simulink model "Vis_CSGO_T_L_NM"  (R2017a)
settings: Solver=FixedStepDiscrete  StartTime=0.0  StopTime=inf  FixedStep=1/250  RelTol=1e-3  EnableMultiTasking=on
StopFcn:
  | AutoStartBatchData=load('session1.mat');AutoStartBatchData=AutoStartBatchData.y;run('AEP_P300_Evaluation')
model workspace (MAT data in the model file):
  cfg_native : struct (value not decoded)
  en_add_channels = 127
  host_ip = 2130706433
  host_port = 50223
  local_ip = 2130706433
  local_port = 50224
  num_en_channels = 32
  num_samples = 4
  sample_rate = 250
  serial_number = 'NR-2018.09.02'
undefined symbols (not defined in the file): groupMap, NR
libraries: gtecHighspeedLib x9, simulink x3, gNautilusLib x1
settings Model: Creator=Holzner  LastModifiedBy=user
settings DataIOCC: LimitDataPoints=on  SaveFormat=Array
settings OptimizationCC: LifeSpan=inf
settings DebuggingCC: UnderspecifiedInitializationDetection=Classic  MergeDetectMultiDrivingBlocksExec=none  SolverPrmCheckMsg=warning  FrameProcessingCompatibilityMsg=none  StateNameClashWarn=warning  SFUnexpectedBacktrackingDiag=warning  SFNoUnconditionalDefaultTransitionDiag=warning  SFExecutionAtInitializationDiag=none
settings HardwareCC: ProdBitPerPointer=32  ProdBitPerSizeT=32  ProdBitPerPtrDiffT=32  ProdLargestAtomicFloat=None  ProdIntDivRoundTo=Undefined  ProdEndianess=Unspecified  ProdWordSize=32  ProdHWDeviceType=32-bit Generic
settings ModelReferenceCC: PropagateSignalLabelsOutOfModel=off
settings GRTTargetCC: TargetLangStandard=C89/C90 (ANSI)  GeneratePreprocessorConditionals=Disable all
settings ConfigComp: CovMetricSettings=dw  CovHtmlReporting=on  CovSaveCumulativeToWorkspaceVar=on  CovSaveSingleToWorkspaceVar=on  CovExternalEMLEnable=off  CovSFcnEnable=off

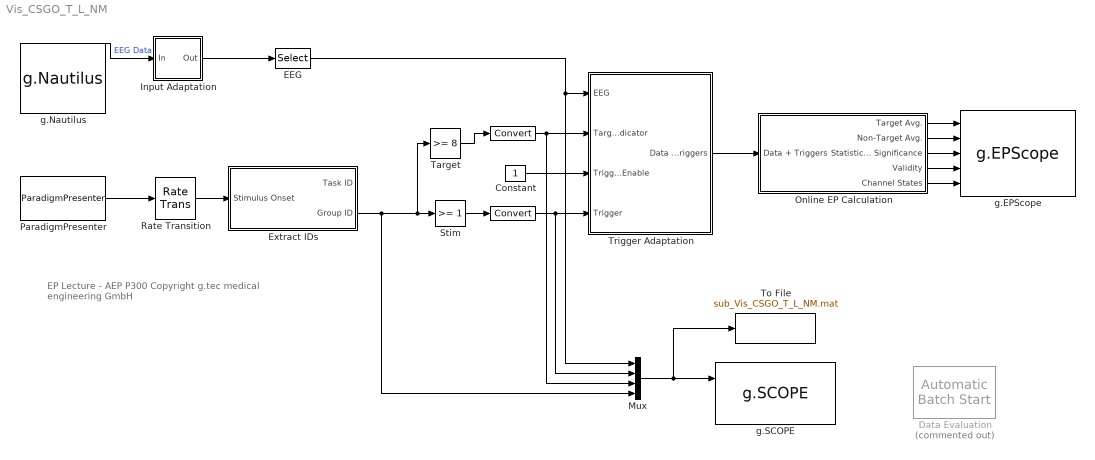
== system Vis_CSGO_T_L_NM ==
  note: EP Lecture - AEP P300
      | Copyright g.tec medical engineering GmbH
  " " : DataTypeConversion
  "  " : DataTypeConversion
  Constant : Constant  SampleTime=-1
  Data Evaluation : gtecHighspeedLib/Automatic  Batch Start  Commented=on  batch2start='AEP_P300_Evaluation'  nameToFileBlock=empty
      settings: SourceProductName=g.tec Highspeed Library
  EEG : Selector  InputPortWidth=32  IndexOptions=Index vector (dialog)  Indices=[1:32]  OutputSizes=1
  Extract IDs : Subsystem
  Input Adaptation : Subsystem
  Mux : Mux
  Online EP Calculation : Subsystem  mask(Online EP Calculation){data_ch_count=32}
      mask prompts: data_ch_count "Number of data channels:"
      mask help:
      | Calculates the target and non-target average of the incoming data and performs statistical significance analysis of target and non-target frames.
      | The data coming in must contain 'Number of data channel' data channels, trigger IDs and target triggers.
  ParadigmPresenter : gtecHighspeedLib/ParadigmPresenter  Priority=2  bufferSize=000001  sampleRateOrig=000250  stimQuantizationUs=002000  paradigmRootFolder=C:\Users\user.T440_IT\Documents\gtec\gtecHS\Examples_can_be_changed\ParadigmPresenter\Sk_CSGO_exp_xml  logLevel=1  paradigmFiles=\Demo\ParadigmPresenterDemo.xml
      settings: SourceProductName=g.tec Highspeed Library
  Rate Transition : RateTransition
  Stim : simulink/Logic and Bit Operations/Compare To Constant  relop=>=  const=1  OutDataTypeStr=boolean
  Target : simulink/Logic and Bit Operations/Compare To Constant  relop=>=  const=8  OutDataTypeStr=boolean
  To File : ToFile  Filename=sub_Vis_CSGO_T_L_NM.mat  MatrixName=y
  Trigger Adaptation : Subsystem
  g.EPScope : gtecHighspeedLib/g.EPScope
      settings: SourceProductName=g.tec Highspeed Library
  g.Nautilus : gNautilusLib/g.Nautilus  Tag=g.Nautilus  Description=Operates a g.Nautilus device and provides acquired data on its outputs.  sample_rate=250  local_ip=2130706433  local_port=50224  host_ip=2130706433  host_port=50223  serial_number=NR-2018.09.02  num_samples=4  num_en_channels=32  add_channels=127
      settings: SourceProductName=g.Nautilus
  g.SCOPE : gtecHighspeedLib/g.SCOPE
      settings: SourceProductName=g.tec Highspeed Library
  wires:
  EEG/1 -> Mux/1, Trigger Adaptation/1(EEG)
  Input Adaptation/1(Out) -> EEG/1
  g.Nautilus/1 -> Input Adaptation/1(In)  "EEG Data"
  Mux/1 -> To File/1, g.SCOPE/1
  Online EP Calculation/1(Target Avg.) -> g.EPScope/1
  Online EP Calculation/2(Non-Target Avg.) -> g.EPScope/2
  Online EP Calculation/3(Statistical Significance) -> g.EPScope/3
  Online EP Calculation/4(Validity) -> g.EPScope/4
  Online EP Calculation/5(Channel States) -> g.EPScope/5
  Trigger Adaptation/1(Data + Triggers) -> Online EP Calculation/1(Data + Triggers)
  ParadigmPresenter/1 -> Rate Transition/1
  Rate Transition/1 -> Extract IDs/1(Stimulus Onset)
  Extract IDs/2(Group ID) -> Target/1, Stim/1, Mux/4
  Target/1 -> " "/1
  Constant/1 -> Trigger Adaptation/3(Trigger Enable)
  "  "/1 -> Mux/2, Trigger Adaptation/4(Trigger)
  Stim/1 -> "  "/1
  " "/1 -> Trigger Adaptation/2(Target Indicator), Mux/3

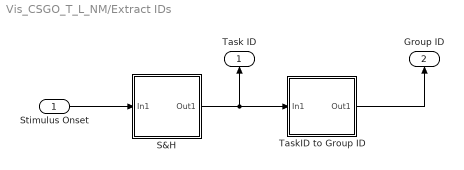
== system Vis_CSGO_T_L_NM/Extract IDs ==
  Stimulus Onset : Inport
  S&H : Subsystem
  TaskID to Group ID : Subsystem  InitFcn=|
      | try
      |   taskInfo = evalin('base','taskInfo');
      |   groupMap = taskInfo.Group;
      | catch ME
      |   clear ME;
      |   error('No paradigm loaded!');
      | end
  Task ID : Outport
  Group ID : Outport  Port=2
  wires:
  TaskID to Group ID/1(Out1) -> Group ID/1
  S&H/1(Out1) -> TaskID to Group ID/1(In1), Task ID/1
  Stimulus Onset/1 -> S&H/1(In1)

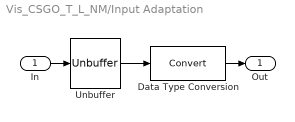
== system Vis_CSGO_T_L_NM/Input Adaptation ==
  In : Inport
  Data Type Conversion : DataTypeConversion
  Unbuffer : Unbuffer
  Out : Outport
  wires:
  In/1 -> Unbuffer/1
  Unbuffer/1 -> Data Type Conversion/1
  Data Type Conversion/1 -> Out/1

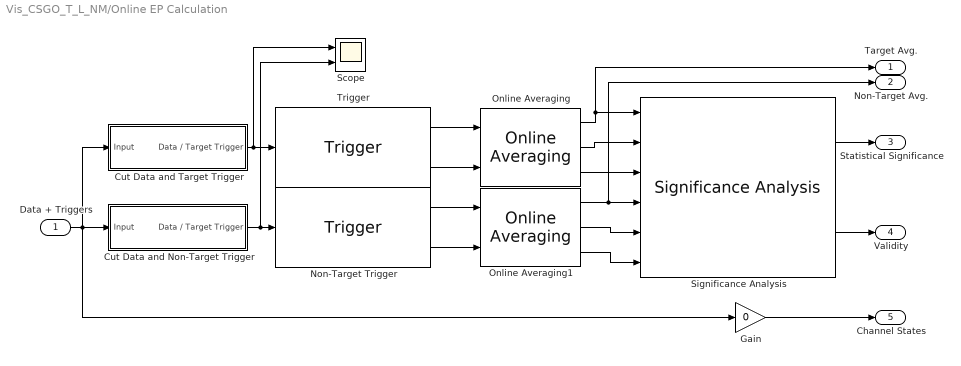
== system Vis_CSGO_T_L_NM/Online EP Calculation ==
  Data + Triggers : Inport
  Cut Data and Non-Target Trigger : Subsystem
  Cut Data and Target Trigger : Subsystem
  Gain : Gain  Gain=0
  Non-Target Trigger : gtecHighspeedLib/Trigger  trigchan=9  edge_select=RISING  edge=0  treshold=1  ext_treshold=off  windowsize=0.7  pretrigger=-0.1  sampletime=1/250  validity_select=STANDARD (global validity flag for all channels)  validity=0
      settings: SourceProductName=g.tec Highspeed Library
  Online Averaging : gtecHighspeedLib/Online Averaging  mode_select=1 - average all data  mode=0  window=10  add_std=on  do_baseline_correction=off  baseline_interval=[0 0]  sampletime=1/250
      settings: SourceProductName=g.tec Highspeed Library
  Online Averaging1 : gtecHighspeedLib/Online Averaging  mode_select=1 - average all data  mode=0  window=10  add_std=on  do_baseline_correction=off  baseline_interval=[0 0]  sampletime=1/250
      settings: SourceProductName=g.tec Highspeed Library
  Scope : Scope  NumInputPorts=2
  Significance Analysis : gtecHighspeedLib/Significance Analysis  sampletime=1/250  pValue_select=4 - 0.95  pValue=3  update_mode_select=1 - any Group  update_mode=0
      settings: SourceProductName=g.tec Highspeed Library
  Trigger : gtecHighspeedLib/Trigger  trigchan=9  edge_select=RISING  edge=0  treshold=1  ext_treshold=off  windowsize=0.7  pretrigger=-0.1  sampletime=1/250  validity_select=STANDARD (global validity flag for all channels)  validity=0
      settings: SourceProductName=g.tec Highspeed Library
  Target Avg. : Outport
  Non-Target Avg. : Outport  Port=2
  Statistical Significance : Outport  Port=3
  Validity : Outport  Port=4
  Channel States : Outport  Port=5
  wires:
  Data + Triggers/1 -> Cut Data and Target Trigger/1(Input), Cut Data and Non-Target Trigger/1(Input), Gain/1
  Online Averaging1/2 -> Significance Analysis/5
  Online Averaging1/3 -> Significance Analysis/6
  Significance Analysis/2 -> Validity/1
  Trigger/2 -> Online Averaging/2
  Trigger/1 -> Online Averaging/1
  Non-Target Trigger/1 -> Online Averaging1/1
  Non-Target Trigger/2 -> Online Averaging1/2
  Online Averaging/1 -> Target Avg./1, Significance Analysis/1
  Online Averaging1/1 -> Significance Analysis/4, Non-Target Avg./1
  Significance Analysis/1 -> Statistical Significance/1
  Gain/1 -> Channel States/1
  Cut Data and Target Trigger/1(Data / Target Trigger) -> Scope/1, Trigger/1
  Cut Data and Non-Target Trigger/1(Data / Target Trigger) -> Scope/2, Non-Target Trigger/1
  Online Averaging/2 -> Significance Analysis/2
  Online Averaging/3 -> Significance Analysis/3

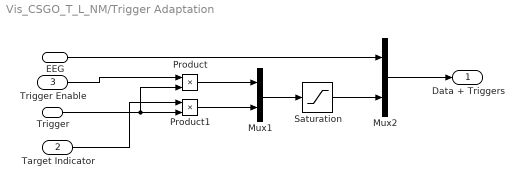
== system Vis_CSGO_T_L_NM/Trigger Adaptation ==
  EEG : Inport
  Target Indicator : Inport  Port=2
  Trigger Enable : Inport  Port=3
  Trigger : Inport  Port=4
  Mux1 : Mux  Inputs=2
  Mux2 : Mux  Inputs=2
  Product : Product
  Product1 : Product
  Saturation : Saturate  UpperLimit=1  LowerLimit=0
  Data + Triggers : Outport
  wires:
  Mux1/1 -> Saturation/1
  Trigger Enable/1 -> Product/1
  Target Indicator/1 -> Product1/1
  Trigger/1 -> Product/2, Product1/2
  Mux2/1 -> Data + Triggers/1
  Saturation/1 -> Mux2/2
  EEG/1 -> Mux2/1
  Product/1 -> Mux1/1
  Product1/1 -> Mux1/2

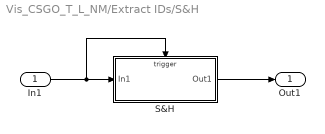
== system Vis_CSGO_T_L_NM/Extract IDs/S&H ==
  In1 : Inport
  S&H : Subsystem  TreatAsAtomicUnit=on
  Out1 : Outport
  wires:
  In1/1 -> S&H/Trigger, S&H/1(In1)
  S&H/1(Out1) -> Out1/1

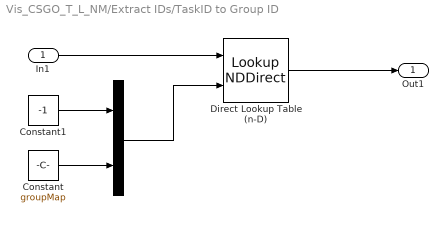
== system Vis_CSGO_T_L_NM/Extract IDs/TaskID to Group ID ==
  In1 : Inport
  " " : Concatenate
  Constant : Constant  Value=groupMap
  Constant1 : Constant  Value=-1
  Direct Lookup Table (n-D) : LookupNDDirect  NumberOfTableDimensions=1  TableIsInput=on  Table=[4 5 ;16 19 ]  DiagnosticForOutOfRangeInput=Error
  Out1 : Outport
  wires:
  Direct Lookup Table (n-D)/1 -> Out1/1
  In1/1 -> Direct Lookup Table (n-D)/1
  Constant/1 -> " "/2
  Constant1/1 -> " "/1
  " "/1 -> Direct Lookup Table (n-D)/2

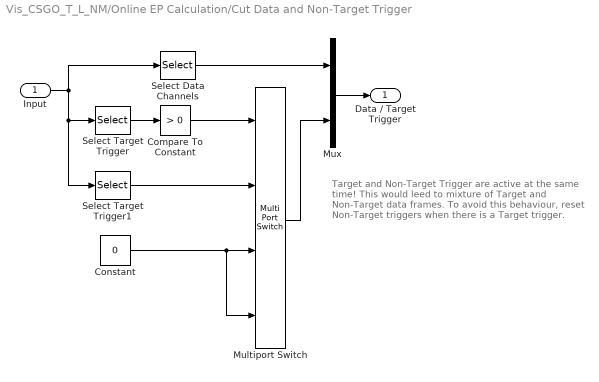
== system Vis_CSGO_T_L_NM/Online EP Calculation/Cut Data and Non-Target Trigger ==
  note: Target and Non-Target Trigger are active at the same time!
      | This would leed to mixture of Target and Non-Target data frames.
      | To avoid this behaviour, reset Non-Target triggers when there is a Target trigger.
  Input : Inport
  Compare To Constant : simulink/Logic and Bit Operations/Compare To Constant  relop=>  const=0  OutDataTypeStr=uint8
  Constant : Constant  Value=0
  Multiport Switch : MultiPortSwitch  DataPortOrder=Zero-based contiguous
  Mux : Mux  Inputs=2
  Select Data Channels : Selector  InputPortWidth=data_ch_count + 2  IndexOptions=Index vector (dialog)  Indices=[1:data_ch_count]  OutputSizes=1
  Select Target Trigger : Selector  InputPortWidth=data_ch_count + 2  IndexOptions=Index vector (dialog)  Indices=data_ch_count+2  OutputSizes=1
  Select Target Trigger1 : Selector  InputPortWidth=data_ch_count + 2  IndexOptions=Index vector (dialog)  Indices=data_ch_count+1  OutputSizes=1
  Data / Target Trigger : Outport
  wires:
  Select Data Channels/1 -> Mux/1
  Mux/1 -> Data / Target Trigger/1
  Input/1 -> Select Data Channels/1, Select Target Trigger1/1, Select Target Trigger/1
  Select Target Trigger/1 -> Compare To Constant/1
  Select Target Trigger1/1 -> Multiport Switch/2
  Constant/1 -> Multiport Switch/4, Multiport Switch/3
  Compare To Constant/1 -> Multiport Switch/1
  Multiport Switch/1 -> Mux/2

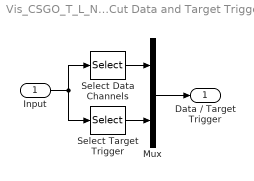
== system Vis_CSGO_T_L_NM/Online EP Calculation/Cut Data and Target Trigger ==
  Input : Inport
  Mux : Mux  Inputs=2
  Select Data Channels : Selector  InputPortWidth=data_ch_count + 2  IndexOptions=Index vector (dialog)  Indices=[1:data_ch_count]  OutputSizes=1
  Select Target Trigger : Selector  InputPortWidth=data_ch_count + 2  IndexOptions=Index vector (dialog)  Indices=data_ch_count+2  OutputSizes=1
  Data / Target Trigger : Outport
  wires:
  Input/1 -> Select Target Trigger/1, Select Data Channels/1
  Select Target Trigger/1 -> Mux/2
  Mux/1 -> Data / Target Trigger/1
  Select Data Channels/1 -> Mux/1

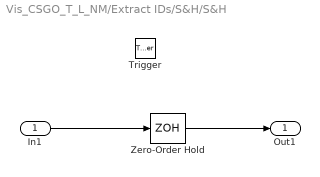
== system Vis_CSGO_T_L_NM/Extract IDs/S&H/S&H ==
  In1 : Inport
  Trigger : TriggerPort  VariantControl=Variant
  Zero-Order Hold : ZeroOrderHold  SampleTime=-1
  Out1 : Outport
  wires:
  In1/1 -> Zero-Order Hold/1
  Zero-Order Hold/1 -> Out1/1
